simulink model "TargetRate"  (R2023b)
settings: Solver=FixedStepAuto  StartTime=0.0  StopTime=7  FixedStep=1e-3  RelTol=1e-3  EnableMultiTasking=on
libraries: dspstat3 x1, frdmk64flib x1
settings Model: SimulationMode=external  ExtModeTrigDuration=5  Creator=Mathew  LastModifiedBy=Mathew
settings DataIOCC: InspectSignalLogs=on
settings OptimizationCC: EnhancedBackFolding=on  PassReuseOutputArgsAs=Individual arguments  ZeroExternalMemoryAtStartup=off  ZeroInternalMemoryAtStartup=off  MaxStackSize=64  OptimizeBlockOrder=speed  DifferentSizesBufferReuse=on  OptimizationCustomize=off  EfficientTunableParamExpr=on
settings DebuggingCC: ParameterTunabilityLossMsg=error
settings HardwareCC: ProdBitPerPointer=32  ProdBitPerSizeT=32  ProdBitPerPtrDiffT=32  ProdLargestAtomicInteger=Long  ProdLargestAtomicFloat=Double  ProdWordSize=32  ProdHWDeviceType=ARM Compatible->ARM Cortex
settings SFSimCC: MATLABDynamicMemAlloc=off
settings RTWCC: Description=Embedded Coder  SystemTargetFile=ert.tlc  HardwareBoard=NXP FRDM-K64F  TLCOptions="-aInlineSetEventsForThisBaseRateFcn=TLC_FALSE -aSuppressMultiTaskScheduler=TLC_FALSE  -aRateBasedStepFcn=0"  TemplateMakefile=ert_default_tmf  Toolchain=GNU Tools for ARM Embedded Processors
settings CodeAppCC: ForceParamTrailComments=on  IgnoreCustomStorageClasses=off  OperatorAnnotations=on  SimulinkDataObjDesc=on  SFDataObjDesc=on  InsertBlockDesc=on
settings ERTTargetCC: ExtMode=on  ExtModeTransport=4  ExtModeMexFile=sendToCommService  ExtModeMexArgs='untitled_restored_from_autosave' 1

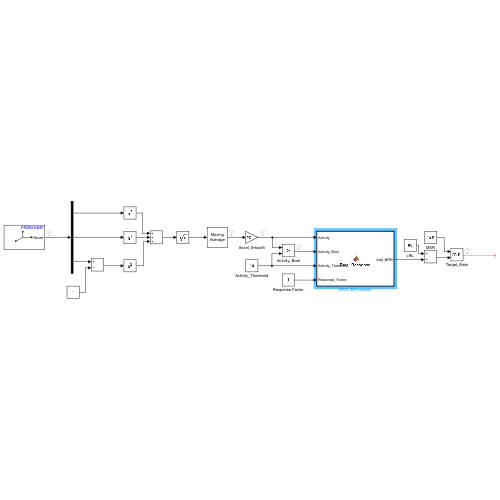
[thumbnail: Simulink's stored preview of the top-level diagram]
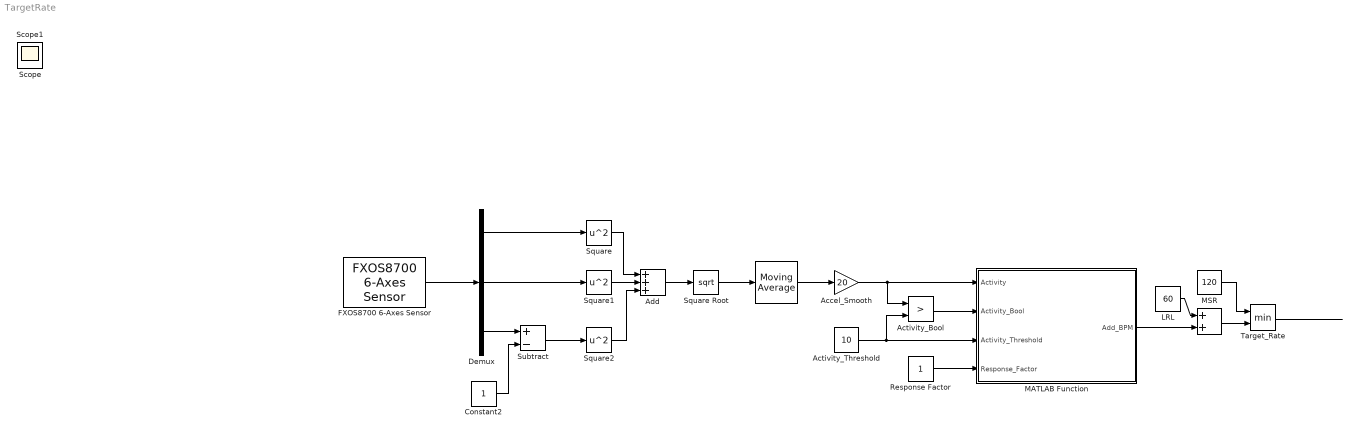
== system TargetRate ==
  " " : dspstat3/Moving Average  Method=Sliding window  ForgettingFactorPort=off  SpecifyWindowLength=on  WindowLength=300  OverlapLength=299  AllowArbitraryInputLength=off  ForgettingFactor=0.9  SimulateUsing=Code generation
  "  " : Sum
  Accel_Smooth : Gain  Gain=20
  Activity_Bool : RelationalOperator  Operator=>  OutDataTypeStr=boolean  RndMeth=Simplest  InputSameDT=off
  Activity_Threshold : Constant  Value=10
  Add : Sum  Inputs=+++
  Constant2 : Constant
  Demux : Demux  Outputs=3
  FXOS8700 6-Axes Sensor : frdmk64flib/FXOS8700 6-Axes Sensor  Activesensor=Accelerometer only  ODR=800Hz  HybridODR=400Hz  Accelfullrange=-4g to +4g  SampleTime=-1
  LRL : Constant  Value=60
  MATLAB Function : MATLAB Function  TreatAsAtomicUnit=on
  MSR : Constant  Value=120
  Response Factor : Constant
  Square : Math  Operator=square
  Square Root : Sqrt
  Square1 : Math  Operator=square
  Square2 : Math  Operator=square
  Subtract : Sum  Inputs=+-
  Target_Rate : MinMax  Inputs=2
  Scope : Scope
  Scope1 : Scope
  wires:
  FXOS8700 6-Axes Sensor/1 -> Demux/1
  Demux/1 -> Square/1
  Demux/2 -> Square1/1
  Square1/1 -> Add/2
  Square/1 -> Add/1
  Square2/1 -> Add/3
  Add/1 -> Square Root/1
  Demux/3 -> Subtract/1
  Subtract/1 -> Square2/1
  Constant2/1 -> Subtract/2
  Square Root/1 -> " "/1
  " "/1 -> Accel_Smooth/1
  Activity_Threshold/1 -> Activity_Bool/2, MATLAB Function/3(Activity_Threshold)
  Accel_Smooth/1 -> Activity_Bool/1, MATLAB Function/1(Activity)
  Activity_Bool/1 -> MATLAB Function/2(Activity_Bool)
  Response Factor/1 -> MATLAB Function/4(Response_Factor)
  MATLAB Function/1(Add_BPM) -> "  "/2
  LRL/1 -> "  "/1
  "  "/1 -> Target_Rate/2
  MSR/1 -> Target_Rate/1
  Target_Rate/1 -> ?

== matlab function TargetRate/MATLAB Function ==
  data: Activity input; Activity_Bool input; Activity_Threshold input; Add_BPM output; Response_Factor input
function Add_BPM = Rate_Response(Activity,Activity_Bool,Activity_Threshold,Response_Factor)

Add_BPM = Activity_Bool*0.3*Response_Factor*(Activity-Activity_Threshold);
